simulink model "Simulacion_Simulink"  (R2023b)
settings: Solver=FixedStepAuto  StartTime=0.0  StopTime=1.01  FixedStep=1e-5  RelTol=1e-3
libraries: fl_lib x7, nesl_utility x4, ee_lib x2
settings Model: Creator=chris  LastModifiedBy=chris

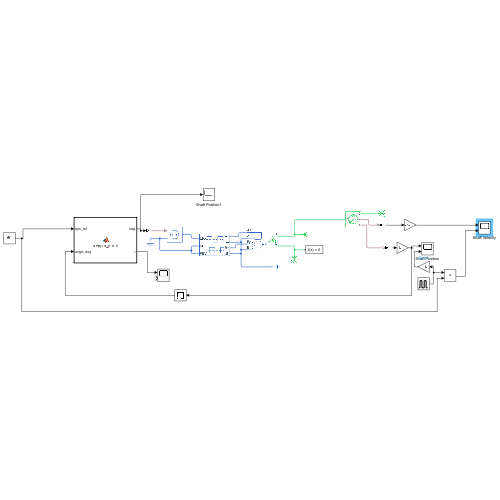
[thumbnail: Simulink's stored preview of the top-level diagram]
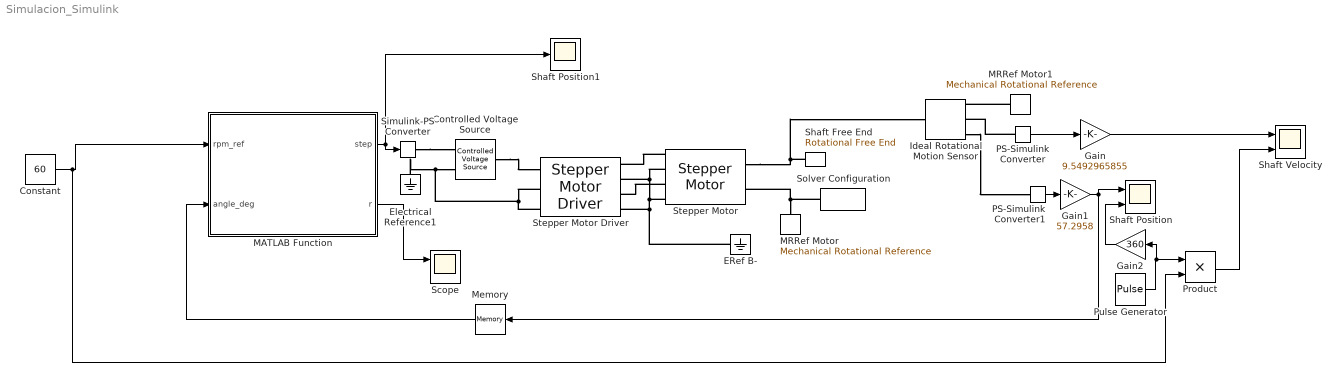
== system Simulacion_Simulink ==
  Constant : Constant  Value=60
  Controlled Voltage Source : fl_lib/Electrical/Electrical Sources/Controlled Voltage Source
  ERef B- : fl_lib/Electrical/Electrical Elements/Electrical Reference
  Electrical Reference1 : fl_lib/Electrical/Electrical Elements/Electrical Reference
  Gain : Gain  Gain=9.5492965855
  Gain1 : Gain  Gain=57.2958
  Gain2 : Gain  Gain=360
  Ideal Rotational Motion Sensor : fl_lib/Mechanical/Mechanical Sensors/Ideal Rotational Motion Sensor  reference=foundation.enum.MeasurementReference.difference  acceleration_port=false  velocity_port=true  position_port=true  wrap_angle=true  offset=0 rad
  MATLAB Function : MATLAB Function  TreatAsAtomicUnit=on
  MRRef Motor : fl_lib/Mechanical/Rotational Elements/Mechanical Rotational Reference
  MRRef Motor1 : fl_lib/Mechanical/Rotational Elements/Mechanical Rotational Reference
  Memory : Memory
  PS-Simulink Converter : nesl_utility/PS-Simulink Converter  PhysicalDomain=network_engine_domain  SubClassName=ps_output  LeftPortType=input  RightPortType=output  PseudoPeriodic=off  Frequencies=[]  VectorFormat=inherit  Unit=inherit  AffineConversion=off
  PS-Simulink Converter1 : nesl_utility/PS-Simulink Converter  PhysicalDomain=network_engine_domain  SubClassName=ps_output  LeftPortType=input  RightPortType=output  PseudoPeriodic=off  Frequencies=[]  VectorFormat=inherit  Unit=inherit  AffineConversion=off
  Product : Product
  Pulse Generator : DiscretePulseGenerator  PulseType=Time based  Period=0.1  PulseWidth=50
  Scope : Scope  NumInputPorts=2
  Shaft Free End : fl_lib/Mechanical/Rotational Elements/Rotational Free End  w_specify=off  w_priority=None  w=0 rad/s  w_nominal_specify=off  w_nominal_unit=rad/s  w_nominal_value=1
  Shaft Position : Scope  NumInputPorts=2
  Shaft Position1 : Scope
  Shaft Velocity : Scope  NumInputPorts=2
  Simulink-PS Converter : nesl_utility/Simulink-PS Converter  PhysicalDomain=network_engine_domain  SubClassName=ps_input  LeftPortType=input  RightPortType=output  PseudoPeriodic=off  Frequencies=[]  NoiseDistribution=none  NoiseParameters=[]  Unit=1  AffineConversion=off  FilteringAndDerivatives=provide  SimscapeFilterOrder=1  InputFilterTimeConstant=0.001  UdotUserProvided=0
  Solver Configuration : nesl_utility/Solver Configuration  PhysicalDomain=network_engine_domain  SubClassName=solver  LeftPortType=input  RightPortType=generic  Tones=[]  Harmonics=[]  SimulateNoise=off  Profile=off  UseLocalSampling=off  EnableSwitchedLinearOptims=on  FrequencyDomain=off  UseCCode=off  RelTol=0.001  AbsTol=1e-06  MinStep=1e-09  ToWorkspace=off  RevertToSquareIcSolve=off  NumHomotopyIterations=100  PhasorMode=off  PhasorModeNumHarmonics=1  ConsistencySolver=NEWTON_FTOL  IndexReductionMethod=DerivativeReplacement  DoDC=off  ResidualTolerance=1e-9  ConsistencyTolSource=GLOBAL  ConsistencyAbsTol=0.001  ConsistencyRelTol=0.001  ConsistencyTolFactor=0.001  UseLocalSolver=off  LocalSolverChoice=NE_BACKWARD_EULER_ADVANCER  ResolveIndetEquations=on  FunctionEvalNumThread=1  LocalSolverSampleTime=.001  DoFixedCost=off  MaxNonlinIter=3  MaxModeIter=2  ComputeImpulses=off  ImpulseIterations=2  LinearAlgebra=auto  LinearAlgebraNumThread=0  EquationFormulation=NE_TIME_EF  DelaysMemoryBudget=1024  AutomaticFiltering=on  FilteringTimeConstant=0.001  PartitionStorageMethod=AS_NEEDED  PartitionMemoryBudget=1024  PartitionMethod=FAST  MultibodyUseLocalSolver=off  MultibodyLocalSolverChoice=ODE1  MultibodyLocalSolverSampleTime=0.001
  Stepper Motor : ee_lib/Electromechanical/Reluctance & Stepper/Stepper Motor  step_or_av=ee.enum.electromech.simulationMode.stepping  Ra=4.1 Ohm  La=4.1e-3 H  Km=0.13 N*m/A  Td=0.02 N*m  Rm=inf Ohm  w_vec=[0, 1000, 3000] rpm  T_vec=[2, 2, 1] N*m  assert_if_slipping=ee.enum.assertAction.none  J_total=1e-4 kg*m^2  max_step_rate=10 Hz  Step=1.8 deg  J=3.08e-6 kg*m^2  B=8.0e-4 N*m*s/rad  speed0=0 rpm  theta0=0 deg  alpha=[.00393, .00393] 1/K  Tmeas=25 degC  Tmeas2=125 degC  T_vec2=[1.7, 1.7, .85] N*m  half_stepping=ee.enum.electromech.steppingModeAveraged.fullStep  thermal_masses=[100, 100] J/K  initial_temperatures=[25, 25] degC  rotor_thermal_mass=50 J/K  rotor_initial_temperature=25 degC  Rm_percent_rotor=90
      settings: InternalSimscapePortConfiguration="{\"Bottom\":[],\"Left\":[{\"id\":\"pA\",\"label\":\"A+\",\"type\":\"foundation.electrical.electrical\"},{\"id\":\"nA\",\"label\":\"A-\",\"type\":\"foundation.electrical.electrical\"},{\"id\":\"pB\",\"label\":\"B+\",\"type\":\"foundation.electrical.electrical\"},{\"id\":\"nB\",\"label\":\"B-\",\"type\":\"foundation.electrical.electrical\"}],\"Right\":[{\"id\":\"R\",\"label\":\"R\",\"type\":\"foundation.mechanical.rotational.rotational\"},{\"id\":\"C\",\"label\":\"C\",\"type\":\"foundation.mechanical.rotational.rotational\"}],\"Top\":[]}"
  Stepper Motor Driver : ee_lib/Electromechanical/Reluctance & Stepper/Stepper Motor Driver  step_or_av=ee.enum.electromech.simulationMode.stepping  step_rate_per_volt=10 Hz/V  Venable=3 V  Vreverse=3 V  supply_ports=ee.enum.supply_ports.hidesupply  Vm=10 V  Vsupply=10 V  half_stepping=ee.enum.electromech.steppingModeAveraged.fullStep  stepping_mode=ee.enum.electromech.steppingMode.microStep  numMicroSteps=32  Im=1 A
      settings: InternalSimscapePortConfiguration="{\"Bottom\":[],\"Left\":[{\"id\":\"ENA\",\"label\":\"ENA\",\"type\":\"foundation.electrical.electrical\"},{\"id\":\"REF\",\"label\":\"REF\",\"type\":\"foundation.electrical.electrical\"},{\"id\":\"REV\",\"label\":\"REV\",\"type\":\"foundation.electrical.electrical\"}],\"Right\":[{\"id\":\"pA\",\"label\":\"A+\",\"type\":\"foundation.electrical.electrical\"},{\"id\":\"nA\",\"label\":\"A-\",\"type\":\"foundation.electrical.electrical\"},{\"id\":\"pB\",\"label\":\"B+\",\"type\":\"foundation.electrical.electrical\"},{\"id\":\"nB\",\"label\":\"B-\",\"type\":\"foundation.electrical.electrical\"}],\"Top\":[]}"
  wires:
  Constant/1 -> Product/2, MATLAB Function/1(rpm_ref)
  Gain/1 -> Shaft Velocity/1
  MATLAB Function/1(step) -> Simulink-PS Converter/1, Shaft Position1/1
  PS-Simulink Converter/1 -> Gain/1
  Memory/1 -> MATLAB Function/2(angle_deg)
  PS-Simulink Converter1/1 -> Gain1/1
  Gain1/1 -> Memory/1, Shaft Position/1
  MATLAB Function/2(r) -> Scope/1
  Pulse Generator/1 -> Gain2/1, Product/1
  Product/1 -> Shaft Velocity/2
  Gain2/1 -> Shaft Position/2
  connections:
  Stepper Motor/LConn1 -- Stepper Motor Driver/RConn1
  Stepper Motor/LConn3 -- Stepper Motor Driver/RConn3
  Stepper Motor/LConn2 -- ERef B-/LConn1 -- Stepper Motor Driver/RConn4 -- Stepper Motor/LConn4 -- Stepper Motor Driver/RConn2
  Shaft Free End/LConn1 -- Ideal Rotational Motion Sensor/LConn1 -- Stepper Motor/RConn1
  MRRef Motor/LConn1 -- Stepper Motor/RConn2 -- Solver Configuration/RConn1
  Electrical Reference1/LConn1 -- Stepper Motor Driver/LConn2 -- Stepper Motor Driver/LConn3 -- Controlled Voltage Source/RConn2
  Simulink-PS Converter/RConn1 -- Controlled Voltage Source/RConn1
  Controlled Voltage Source/LConn1 -- Stepper Motor Driver/LConn1
  MRRef Motor1/LConn1 -- Ideal Rotational Motion Sensor/RConn1
  PS-Simulink Converter/LConn1 -- Ideal Rotational Motion Sensor/RConn2
  Ideal Rotational Motion Sensor/RConn3 -- PS-Simulink Converter1/LConn1

== matlab function Simulacion_Simulink/MATLAB Function ==
  settings: updateMethod=DISCRETE
  data: rpm_ref input; step output; angle_deg input; r output
function [step, r] = stepper_pulse(rpm_ref, angle_deg)
% stepper_pulse - PID cada 50 ms (usa ángulo en grados), STEP/PWM con alta resolución
% Entradas:
%   rpm_ref   : referencia en RPM
%   angle_deg : medida absoluta del ángulo en grados (0..360)
% Salida:
%   step      : señal STEP 0..3.3 V

Ts_pwm = 1e-5;  % resolución de la señal STEP (1e-5 s = 10 us)
Ts_pid = 0.05;  % 50 ms para actualizar el PID

persistent count state integral prev_error t_pid pid_output prev_angle_deg

if isempty(count)
    count = 0;
    state = 0;
    integral = 0;
    prev_error = 0;
    t_pid = 0;
    pid_output = 0;
    prev_angle_deg = angle_deg; % inicializa con la primera medición
end

% ---------------------------
% Actualización del PID cada Ts_pid
% ---------------------------
t_pid = t_pid + Ts_pwm;
if t_pid >= Ts_pid
    % --- calcular delta de ángulo con corrección de wrap-around (±180°) ---
    delta_deg = angle_deg - prev_angle_deg;
    % corregir salto por pasar 360->0 o 0->360
    % Asegurarse de que delta sea positivo
    if delta_deg < 0
        delta_deg = delta_deg + 360;
    end

    % velocidad medida en RPM:
    % delta_deg [deg] en intervalo Ts_pid [s]
    % rpm = (delta_deg / 360) [rev] / Ts_pid [s] * 60 [s/min]
    omega_rpm = (delta_deg / 360) / Ts_pid * 60;
    % alternativa simplificada: omega_rpm = delta_deg * (1/(6*Ts_pid));

    % PID (ganancias iniciales sugeridas)
    Kp = 0.04;
    Ki = 0.004;
    Kd = 0.0002;

    error = rpm_ref - omega_rpm;

    derivative = (error - prev_error) / Ts_pid;
    integral = integral + error * Ts_pid;

    pid_output = Kp*error + Ki*integral + Kd*derivative;

    prev_error = error;
    prev_angle_deg = angle_deg;   % actualizar ángulo previo para la próxima medición

    % --- saturación de r (limitar la acción del controlador) ---
    r_unsat = rpm_ref + pid_output;
    r_min = 0.8*rpm_ref;
    r_max = 1.2*rpm_ref;
    if rpm_ref == 0
        r_min = 0;
        r_max = max(50, rpm_ref + 100); % caso arbitrario para referencia 0
    end
    r_sat = min(max(r_unsat, r_min), r_max);

    % Anti-windup simple: si saturó, deshacer la última integración
    if r_sat ~= r_unsat
        integral = integral - error * Ts_pid;
        pid_output = r_sat - rpm_ref;
    else
        pid_output = r_unsat - rpm_ref;
    end

    t_pid = t_pid - Ts_pid; % conservar residuo de tiempo en caso de Ts_pwm no dividir exacto
end

% ---------------------------
% Generación STEP/PWM (alta resolución)
% ---------------------------
r = rpm_ref + pid_output;   % velocidad objetivo usada por el generador de pulsos
if ~(r > 0)
    step = 0;
    half_period_us=0;
    return;
end

spb = 200; ms = 32;
totalSteps = spb * ms;
period_us = 60000000 / (totalSteps * r);
half_period_us = period_us / 2;

half_samples = max(round(half_period_us * 1e-6 / Ts_pwm), 1);

count = count + 1;
if count >= half_samples
    state = 1 - state; % toggle 0/1
    count = 0;
end

step = 3.3 * state;
end
